simulink model "Maglev_PD_Gravity_2021b"  (R2021b)
settings: Solver=VariableStepAuto  StartTime=0.0  StopTime=50  RelTol=1e-3
values from neighbouring files (symbols this model uses):
  cr = 700    [datasheet.m]    (also in setup.m)
  d0 = 14    [LQRsetup.m]    (also in PIDsetup.m; datasheet.m = 0.01228; setup.m = 0.01228)
  k = u0*As*(N^2)    (= 0.000836467893574)    [datasheet.m]    (also in setup.m)
  Kp_I = 250    [datasheet.m]    (also in setup.m = 3000)
  Lfe = 0.2781    [datasheet.m]    (also in setup.m)
  m = 0.83474    [LQRgen.m]    (also in LQRsetup.m; PIDsetup.m; datasheet.m; setup.m)
  R = tf([K*Lmax, K*R], [1 0])    [ElecTFanalysis.m]    (also in L.m = 3.7; LQRgen.m = 1; LQRsetup.m = 1; datasheet.m = 3.7)
libraries: cstblocks x2, slpidlib x1
settings Model: Creator=dfigu  LastModifiedBy=ricca

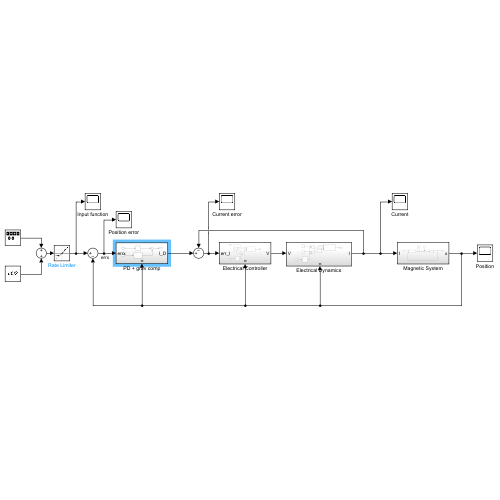
[thumbnail: Simulink's stored preview of the top-level diagram]
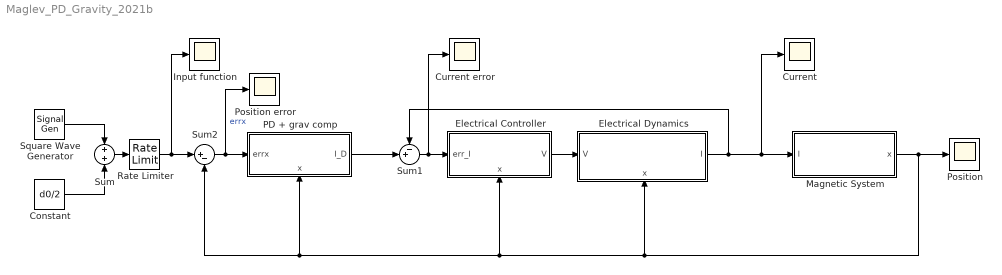
== system Maglev_PD_Gravity_2021b ==
  Constant : Constant  Value=d0/2
  Current : Scope
  Current error : Scope
  Electrical Controller : Subsystem
      settings: PortSchema="{\"entries\":[{\"content\":{\"sides\":[{\"content\":{\"connectorIds\":[\"In1\"]},\"type\":\"ConnectorPlacement.EquallySpacedRectSide\",\"uuid\":\"3fdb2aee-0f97-4270-a8d8-9bae33eb88d8\"},{\"content\":{\"connectorIds\":[\"Out1\"],\"side\":\"RIGHT\"},\"type\":\"ConnectorPlacement.EquallySpacedRectSide\",\"uuid\":\"1e882846-237e-4335-8f0f-7b0630d47a70\"},{\"content\":{\"connectorIds\":[],\"side\":\"TOP\"},\"type\":\"ConnectorPlacement.EquallySpacedRectSide\",\"uuid\":\"058d3edc-cae6-48db-a5f0-79976918138f\"},{\"content\":{\"connectorIds\":[\"In2\"],\"side\":\"BOTTOM\"},\"type\":\"ConnectorPlacement.EquallySpacedRectSide\",\"uuid\":\"8b25cdbb-e979-4478-9946-b7a1ad4d4563\"}]},\"type\":\"ConnectorPlacement.EquallySpacedConnector\",\"uuid\":\"e66bf500-41d2-4dc7-9a99-4f4f01c47e0d\"}],\"packageUris\":[\"http://schema.mathworks.com/mf0/Connector/R2020b\"],\"version\":\"1.0\"}"
  Electrical Dynamics : Subsystem
      settings: PortSchema="{\"entries\":[{\"content\":{\"sides\":[{\"content\":{\"connectorIds\":[\"In1\"]},\"type\":\"ConnectorPlacement.EquallySpacedRectSide\",\"uuid\":\"3fdb2aee-0f97-4270-a8d8-9bae33eb88d8\"},{\"content\":{\"connectorIds\":[\"Out1\"],\"side\":\"RIGHT\"},\"type\":\"ConnectorPlacement.EquallySpacedRectSide\",\"uuid\":\"1e882846-237e-4335-8f0f-7b0630d47a70\"},{\"content\":{\"connectorIds\":[],\"side\":\"TOP\"},\"type\":\"ConnectorPlacement.EquallySpacedRectSide\",\"uuid\":\"058d3edc-cae6-48db-a5f0-79976918138f\"},{\"content\":{\"connectorIds\":[\"In2\"],\"side\":\"BOTTOM\"},\"type\":\"ConnectorPlacement.EquallySpacedRectSide\",\"uuid\":\"24ad4b22-37ce-44f4-8c66-526992c2d85a\"}]},\"type\":\"ConnectorPlacement.EquallySpacedConnector\",\"uuid\":\"e66bf500-41d2-4dc7-9a99-4f4f01c47e0d\"}],\"packageUris\":[\"http://schema.mathworks.com/mf0/Connector/R2020b\"],\"version\":\"1.0\"}"
  Input function : Scope
  Magnetic System : Subsystem
  PD + grav comp : Subsystem
      settings: PortSchema="{\"entries\":[{\"content\":{\"sides\":[{\"content\":{\"connectorIds\":[\"In1\"]},\"type\":\"ConnectorPlacement.EquallySpacedRectSide\",\"uuid\":\"3fdb2aee-0f97-4270-a8d8-9bae33eb88d8\"},{\"content\":{\"connectorIds\":[\"Out1\"],\"side\":\"RIGHT\"},\"type\":\"ConnectorPlacement.EquallySpacedRectSide\",\"uuid\":\"1e882846-237e-4335-8f0f-7b0630d47a70\"},{\"content\":{\"connectorIds\":[],\"side\":\"TOP\"},\"type\":\"ConnectorPlacement.EquallySpacedRectSide\",\"uuid\":\"058d3edc-cae6-48db-a5f0-79976918138f\"},{\"content\":{\"connectorIds\":[\"In2\"],\"side\":\"BOTTOM\"},\"type\":\"ConnectorPlacement.EquallySpacedRectSide\",\"uuid\":\"c1784ea1-d60e-42df-b11a-c0a12452713b\"}]},\"type\":\"ConnectorPlacement.EquallySpacedConnector\",\"uuid\":\"e66bf500-41d2-4dc7-9a99-4f4f01c47e0d\"}],\"packageUris\":[\"http://schema.mathworks.com/mf0/Connector/R2020b\"],\"version\":\"1.0\"}"
  Position : Scope
  Position error : Scope
  Rate Limiter : RateLimiter  RisingSlewLimit=0.01  FallingSlewLimit=-0.01  SampleTimeMode=inherited
  Square Wave Generator : SignalGenerator  WaveForm=square  Amplitude=d0/4  Frequency=0.1
  Sum : Sum  Inputs=+|+
  Sum1 : Sum  Inputs=-+|
  Sum2 : Sum  Inputs=|+-
  wires:
  Electrical Dynamics/1(I) -> Current/1, Magnetic System/1(I), Sum1/1
  Sum1/1 -> Current error/1, Electrical Controller/1(err_I)
  Electrical Controller/1(V) -> Electrical Dynamics/1(V)
  PD + grav comp/1(I_D) -> Sum1/2
  Magnetic System/1(x) -> Electrical Dynamics/2(x), Electrical Controller/2(x), Sum2/2, PD + grav comp/2(x), Position/1
  Sum2/1 -> Position error/1, PD + grav comp/1(errx)  "errx"
  Square Wave Generator/1 -> Sum/1
  Constant/1 -> Sum/2
  Sum/1 -> Rate Limiter/1
  Rate Limiter/1 -> Input function/1, Sum2/1

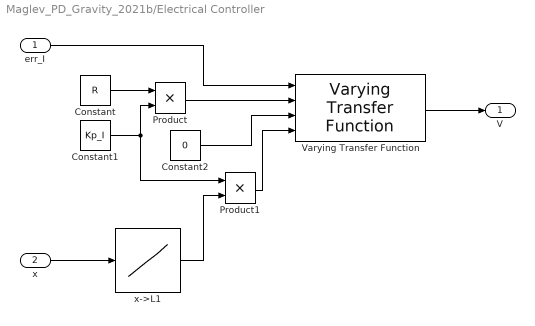
== system Maglev_PD_Gravity_2021b/Electrical Controller ==
  err_I : Inport
  x : Inport  Port=2
  Constant : Constant  Value=R
  Constant1 : Constant  Value=Kp_I
  Constant2 : Constant  Value=0
  Product : Product
  Product1 : Product
  Varying Transfer Function : cstblocks/Linear Parameter Varying/Varying Transfer Function  N=1
  x->L1 : Lookup_n-D  NumberOfTableDimensions=1  BreakpointsForDimension1=[0,0.002,0.007,0.0096,0.011,0.0143,0.01445]  Table=[0.1086,0.114,0.129,0.148,0.165,0.250,0.350]  InternalRulePriority=Speed  RndMeth=Simplest  InputSameDT=on
  V : Outport
  wires:
  x/1 -> x->L1/1
  err_I/1 -> Varying Transfer Function/1
  Varying Transfer Function/1 -> V/1
  Product/1 -> Varying Transfer Function/2
  Constant/1 -> Product/1
  Constant1/1 -> Product1/1, Product/2
  Constant2/1 -> Varying Transfer Function/3
  Product1/1 -> Varying Transfer Function/4
  x->L1/1 -> Product1/2

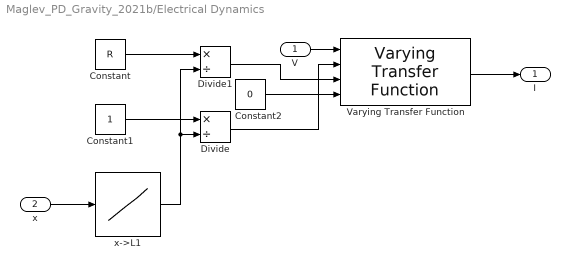
== system Maglev_PD_Gravity_2021b/Electrical Dynamics ==
  V : Inport
  x : Inport  Port=2
  Constant : Constant  Value=R
  Constant1 : Constant
  Constant2 : Constant  Value=0
  Divide : Product  Inputs=*/
  Divide1 : Product  Inputs=*/
  Varying Transfer Function : cstblocks/Linear Parameter Varying/Varying Transfer Function  N=1
  x->L1 : Lookup_n-D  NumberOfTableDimensions=1  BreakpointsForDimension1=[0,0.002,0.007,0.0096,0.011,0.0143,0.01445]  Table=[0.1086,0.114,0.129,0.148,0.165,0.250,0.350]  InternalRulePriority=Speed  RndMeth=Simplest  InputSameDT=on
  I : Outport
  wires:
  V/1 -> Varying Transfer Function/1
  x/1 -> x->L1/1
  Constant1/1 -> Divide/1
  x->L1/1 -> Divide1/2, Divide/2
  Divide/1 -> Varying Transfer Function/2
  Constant/1 -> Divide1/1
  Divide1/1 -> Varying Transfer Function/3
  Constant2/1 -> Varying Transfer Function/4
  Varying Transfer Function/1 -> I/1

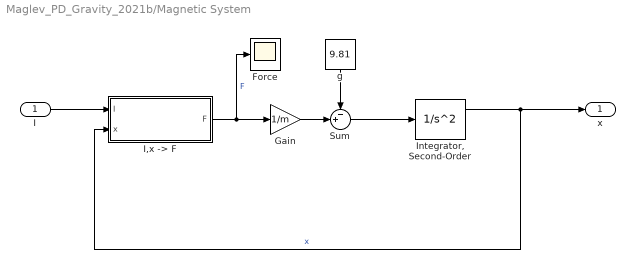
== system Maglev_PD_Gravity_2021b/Magnetic System ==
  I : Inport
  Force : Scope
  Gain : Gain  Gain=1/m
  "I,x -> F" : Subsystem
  "Integrator, Second-Order" : SecondOrderIntegrator  ICX=x0  LimitX=on  UpperLimitX=d0  LowerLimitX=0
  Sum : Sum  Inputs=-+|
  g : Constant  Value=9.81
  x : Outport
  wires:
  "I,x -> F"/1(F) -> Force/1, Gain/1  "F"
  Gain/1 -> Sum/2
  Sum/1 -> "Integrator, Second-Order"/1
  "Integrator, Second-Order"/1 -> x/1, "I,x -> F"/2(x)  "x"
  g/1 -> Sum/1
  I/1 -> "I,x -> F"/1(I)

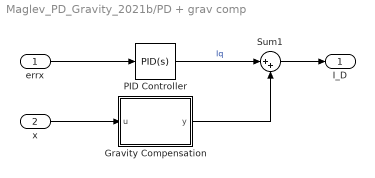
== system Maglev_PD_Gravity_2021b/PD + grav comp ==
  errx : Inport
  x : Inport  Port=2
  Gravity Compensation : MATLAB Function  TreatAsAtomicUnit=on
  PID Controller : slpidlib/PID Controller  Controller=PID  Form=Parallel  TimeDomain=Continuous-time  UseExternalTs=off  SampleTime=-1  IntegratorMethod=Forward Euler  FilterMethod=Forward Euler  ControllerParametersSource=internal  P=0.2  I=0  D=5  UseFilter=on  N=100  TunerSelectOption=Transfer Function Based (PID Tuner App)  InitialConditionSource=internal  InitialConditionForIntegrator=0  InitialConditionForFilter=0  DifferentiatorICPrevScaledInput=0  ExternalReset=none  TrackingMode=off  Kt=1  LimitOutput=on  SatLimitsSource=internal  UpperSaturationLimit=inf  LowerSaturationLimit=-inf  LinearizeAsGain=on  AntiWindupMode=back-calculation  Kb=1000  POutMin=[]  POutMax=[]  IOutMin=[]  IOutMax=[]  DOutMin=[]  DOutMax=[]  NOutMin=[]  NOutMax=[]  SumOutMin=[]  SumOutMax=[]  SaturationOutMin=[]  SaturationOutMax=[]  PParamMin=[]  PParamMax=[]  IParamMin=[]  IParamMax=[]  DParamMin=[]  DParamMax=[]  NParamMin=[]  NParamMax=[]  KbParamMin=[]  KbParamMax=[]  KtParamMin=[]  KtParamMax=[]  KbOutMin=[]  KbOutMax=[]  KtOutMin=[]  KtOutMax=[]  IntegratorOutMin=[]  IntegratorOutMax=[]  FilterOutMin=[]  FilterOutMax=[]  SumI1OutMin=[]  SumI1OutMax=[]  SumI2OutMin=[]  SumI2OutMax=[]  SumI3OutMin=[]  SumI3OutMax=[]  SumI4OutMin=[]  SumI4OutMax=[]  SumDOutMin=[]  SumDOutMax=[]  DifferentiatorOutMin=[]  DifferentiatorOutMax=[]  FilterDiffOutCoefMin=[]  FilterDiffOutCoefMax=[]  ReciprocalOutMin=[]  ReciprocalOutMax=[]  SumDenOutMin=[]  SumDenOutMax=[]  SumNumOutMin=[]  SumNumOutMax=[]  DivideOutMin=[]  DivideOutMax=[]  UdiffTsProdOutMin=[]  UdiffTsProdOutMax=[]  NTsProdOutMin=[]  NTsProdOutMax=[]  UintegralTsProdOutMin=[]  UintegralTsProdOutMax=[]  UngainTsProdOutMin=[]  UngainTsProdOutMax=[]  IntegratorContinuousStateAttributes=''  IntegratorStateMustResolveToSignalObject=off  IntegratorRTWStateStorageClass=Auto  FilterContinuousStateAttributes=''  FilterStateMustResolveToSignalObject=off  FilterRTWStateStorageClass=Auto  ParallelPVariant=InternalParameters  IdealPVariant=Disabled  IVariant=InternalParameters  DVariant=InternalParameters  IntegratorVariant=Continuous  SatVariant=Enabled  AWVariant=BackCalculation  PCopyVariant=Disabled  TRVariant=Disabled  FdbkBlocksVariant=Forward  IdealPFdbkVariant=Disabled  SatFdbkVariant=Disabled  DerivativeFilterVariant=ContFilter  NVariant=InternalParameters  NCopyVariant=Disabled  FilterICVariant=InternalICsFilter  IntegratorICVariant=InternalICs  ExternalResetVariant=Disabled  TRSumVariant=Passthrough  SumFdbkVariant=Disabled  SumVariant=Sum_PID  TsampFilterVariant=InternalTs  TsampNgainVariant=Passthrough  TsampIntegralVariant=Passthrough  ExternalSaturationOutDataTypeStr=Inherit: Same as second input
  Sum1 : Sum  Inputs=|++
  I_D : Outport
  wires:
  Sum1/1 -> I_D/1
  PID Controller/1 -> Sum1/1  "Iq"
  x/1 -> Gravity Compensation/1(u)
  Gravity Compensation/1(y) -> Sum1/2
  errx/1 -> PID Controller/1

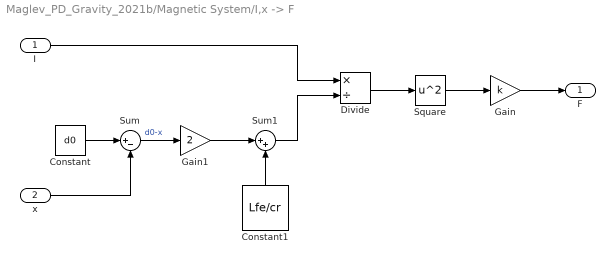
== system Maglev_PD_Gravity_2021b/Magnetic System/I,x -> F ==
  I : Inport
  x : Inport  Port=2
  Constant : Constant  Value=d0
  Constant1 : Constant  Value=Lfe/cr
  Divide : Product  Inputs=*/
  Gain : Gain  Gain=k
  Gain1 : Gain  Gain=2
  Square : Math  Operator=square  SaturateOnIntegerOverflow=on
  Sum : Sum  Inputs=|+-
  Sum1 : Sum  Inputs=|++
  F : Outport
  wires:
  Gain/1 -> F/1
  Constant/1 -> Sum/1
  x/1 -> Sum/2
  Sum/1 -> Gain1/1  "d0-x"
  Gain1/1 -> Sum1/1
  Constant1/1 -> Sum1/2
  Sum1/1 -> Divide/2
  Square/1 -> Gain/1
  Divide/1 -> Square/1
  I/1 -> Divide/1

== matlab function Maglev_PD_Gravity_2021b/PD + grav comp/Gravity Compensation ==
  data: u input; y output
function y = fcn(u)
m = 0.83474;      %mass
N = 860;    %spires
Lb = 0.03;  %width
Pb = 0.03;  %depth
d0 = 0.01228;     %delta0
u0 = 4*pi*10^(-7);  %permeabilità vuoto
cr = 700;   %coefficiente magnetismo ferro
Lfe = 0.2781; %Lunghezza circuito ferro

As = Lb*Pb;
k = u0*As*(N^2);
y = sqrt((m*9.81*(Lfe/cr+2*(d0-u))^2)/(k));
